simulink model "PRCT3_MTras"  (R2022b)
settings: Solver=VariableStepAuto  StartTime=0.0  StopTime=10.0  RelTol=1e-3
values from neighbouring files (symbols this model uses):
  b1 = 1000    [PRCT3.m]    (also in PRCT3P.m)
  k1 = 16182    [PRCT3.m]    (also in PRCT3P.m)
  k2 = 19000    [PRCT3.m]    (also in PRCT3P.m)
  m1 = 290    [PRCT3.m]    (also in PRCT3P.m)
  m2 = 59    [PRCT3.m]    (also in PRCT3P.m)
settings Model: Creator=josel  LastModifiedBy=josel

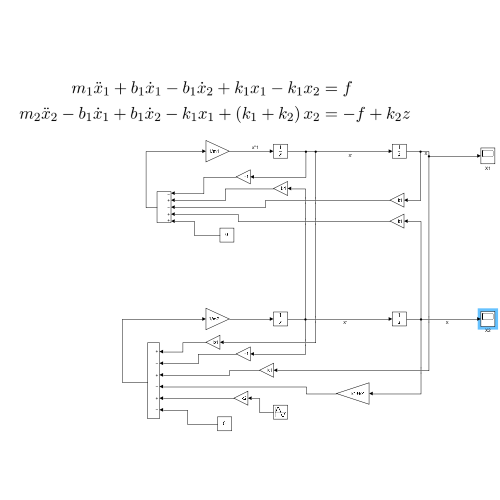
[thumbnail: Simulink's stored preview of the top-level diagram]
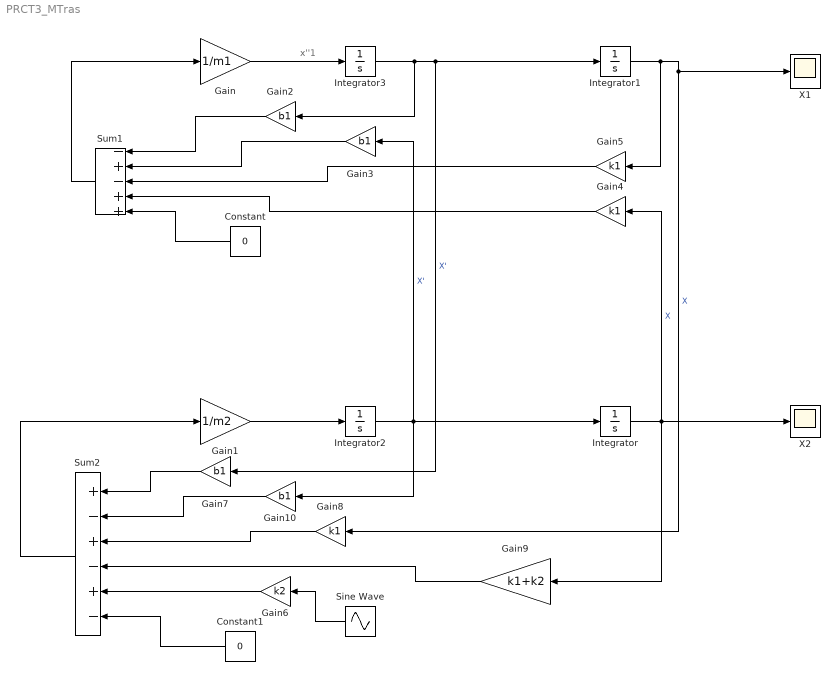
== system PRCT3_MTras ==
  note: x''1
  Constant : Constant  Value=0
  Constant1 : Constant  Value=0
  Gain : Gain  Gain=1/m1
  Gain1 : Gain  Gain=1/m2
  Gain{2..3,7,10} (4 alike) : Gain  Gain=b1
  Gain4 : Gain  Gain=k1
  Gain5 : Gain  Gain=k1
  Gain6 : Gain  Gain=k2
  Gain8 : Gain  Gain=k1
  Gain9 : Gain  Gain=k1+k2
  Integrator{,1..3} (4 alike) : Integrator
  Sine Wave : Sin  Amplitude=0.05  Frequency=0.5*pi  SampleTime=0
  Sum1 : Sum  Inputs=-+-++
  Sum2 : Sum  Inputs=+-+-+-
  X1 : Scope
  X2 : Scope
  wires:
  Gain/1 -> Integrator3/1
  Integrator3/1 -> Gain7/1, Integrator1/1, Gain2/1  "X'"
  Gain1/1 -> Integrator2/1
  Integrator2/1 -> Gain10/1, Integrator/1, Gain3/1  "X'"
  Integrator/1 -> Gain9/1, Gain4/1, X2/1  "X"
  Integrator1/1 -> Gain5/1, Gain8/1, X1/1  "X"
  Sum1/1 -> Gain/1
  Gain2/1 -> Sum1/1
  Gain3/1 -> Sum1/2
  Gain5/1 -> Sum1/3
  Gain4/1 -> Sum1/4
  Sum2/1 -> Gain1/1
  Sine Wave/1 -> Gain6/1
  Constant/1 -> Sum1/5
  Gain6/1 -> Sum2/5
  Constant1/1 -> Sum2/6
  Gain7/1 -> Sum2/1
  Gain10/1 -> Sum2/2
  Gain8/1 -> Sum2/3
  Gain9/1 -> Sum2/4
